simulink subsystem "Day2_Scenario_1"  (R2024a)
settings: Solver=VariableStepAuto  StartTime=0.0  StopTime=10.0  RelTol=1e-3
libraries: CarMaker4SL x2
settings Model: Creator=junhyung.cha  LastModifiedBy=pc

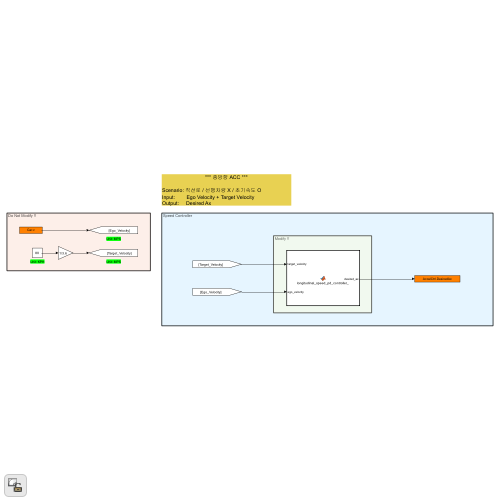
[thumbnail: Simulink's stored preview of the top-level diagram]
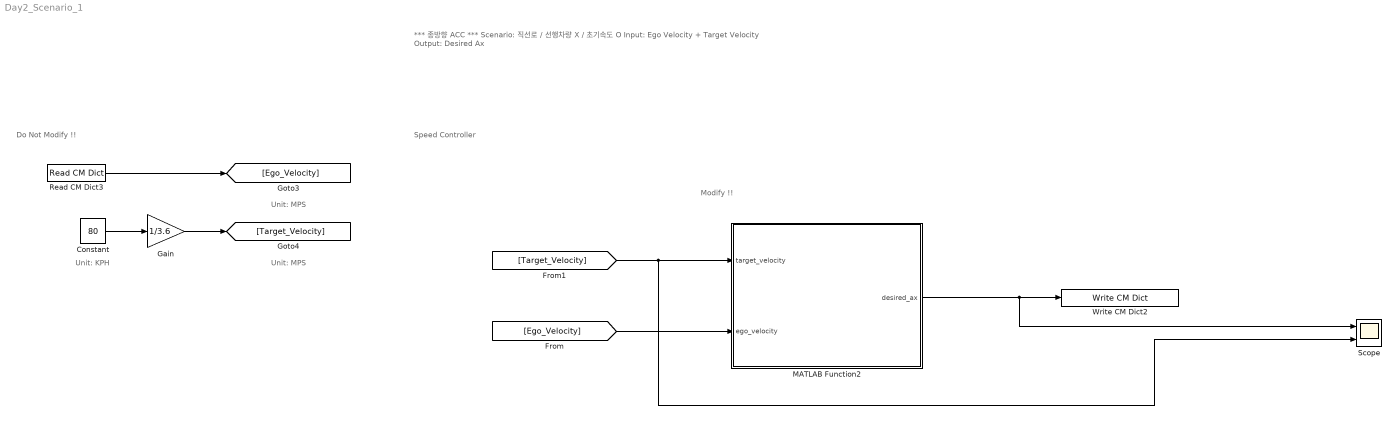
== system Day2_Scenario_1 ==
  note: Unit: KPH
  note: *** 종방향 ACC ***
      |
      | Scenario: 직선로 / 선행차량 X / 초기속도 O
      | Input: Ego Velocity + Target Velocity
      | Output: Desired Ax
  note: Do Not Modify !!
  note: Modify !!
  note: Speed Controller
  note: Unit: MPS
  note: Unit: MPS
  Constant : Constant  Value=80
  Gain : Gain  Gain=1/3.6
  MATLAB Function2 : MATLAB Function  TreatAsAtomicUnit=on
  Read CM Dict3 : CarMaker4SL/Read CM Dict  xname=Car.v  xsync=off  xstime=Inherited
  Scope : Scope  NumInputPorts=2
  Write CM Dict2 : CarMaker4SL/Write CM Dict  xname=AccelCtrl.DesiredAx  xsync=off
  wires:
  MATLAB Function2/1(desired_ax) -> Write CM Dict2/1, Scope/1
  [Target_Velocity] -> MATLAB Function2/1(target_velocity), Scope/2
  Constant/1 -> Gain/1
  [Ego_Velocity] -> MATLAB Function2/2(ego_velocity)
  Read CM Dict3/1 -> [Ego_Velocity]
  Gain/1 -> [Target_Velocity]

== matlab function Day2_Scenario_1/MATLAB Function2 ==
  settings: updateMethod=DISCRETE  sampleTime=0.05
  data: target_velocity input; desired_ax output; ego_velocity input
function desired_ax = longitudinal_speed_pd_controller_(target_velocity, ego_velocity)
%#codegen

    % PD 제어기 게인
    Kp = 1.5;   % 비례 게인
    Kd = 0.2;   % 미분 게인
    dt = 0.05;  % 샘플링 시간 (초), 모델 설정에 맞게 조정

    % 속도 오차 계산
    error = target_velocity - ego_velocity;

    % 이전 오차 저장을 위한 persistent 변수
    persistent prev_error
    if isempty(prev_error)
        prev_error = 0;
    end

    % 오차의 미분 계산
    derivative = (error - prev_error) / dt;

    % PD 제어기 계산
    desired_ax = Kp * error + Kd * derivative;

    % 이전 오차 업데이트
    prev_error = error;
end
